simulink model "TwoDOF"  (R2021b)
settings: Solver=VariableStepAuto  StartTime=0.0  StopTime=7  RelTol=1e-3
values from neighbouring files (symbols this model uses):
  Ask = [0 1 0 0 ... (first row only)    [H_inf_ctrl.m]
  Bsk = [0 0 0 0 ... (first row only)    [H_inf_ctrl.m]
  c = 40e3    (= 40000)    [H_inf_ctrl.m]
  c_p = 0.8    [H_inf_ctrl.m]
  c_s = 0.05    [H_inf_ctrl.m]
  c_x = 3300000    [H_inf_ctrl.m]
  c_z = 1000000    [H_inf_ctrl.m]
  Csk = [0 1 0 0 ... (first row only)    [H_inf_ctrl.m]
  Dsk = zeros(2,4)    [H_inf_ctrl.m]
  j = 700e3    (= 700000)    [H_inf_ctrl.m]
  k = 2*300e3    (= 600000)    [H_inf_ctrl.m]
  k_p = 6.32    [H_inf_ctrl.m]
  k_s = 0.0632    [H_inf_ctrl.m]
  L = 6    [H_inf_ctrl.m]
  m = 22000    [H_inf_ctrl.m]
  m_p = 0.16    [H_inf_ctrl.m]
  m_s = 0.16    [H_inf_ctrl.m]
  T = 0.1    [H_inf_ctrl.m]    (also in OneDOF.m = 1.5; PID_Controller.m = 1.5)
  w_n = sqrt(k_p/m_p)    [H_inf_ctrl.m]
undefined symbols (not defined in the file or in its folder): K
settings Model: Creator=thomasperrein  LastModifiedBy=thomasperrein

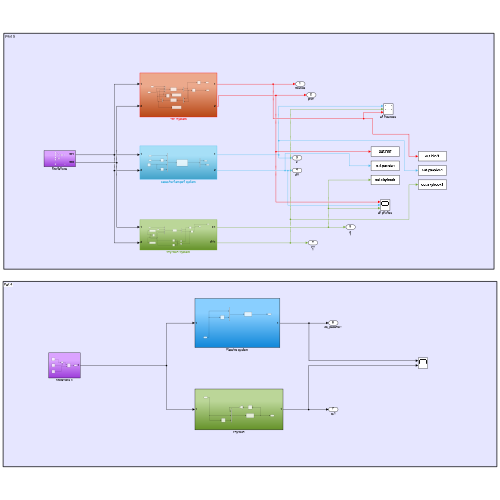
[thumbnail: Simulink's stored preview of the top-level diagram]
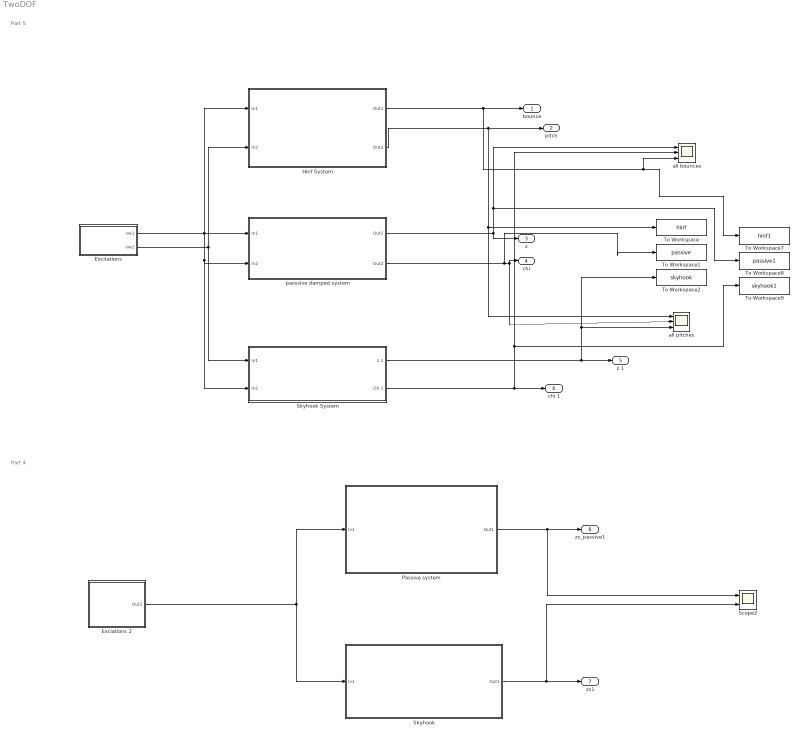
== system TwoDOF ==
  note: Part 4
  note: Part 5
  Exciations 2 : Subsystem
  Excitations : Subsystem
  Hinf System : Subsystem
  Passive system : Subsystem
  Scope2 : Scope  NumInputPorts=2
  Skyhook : Subsystem
  Skyhook System : Subsystem
  To Workspace : ToWorkspace  VariableName=hinf  SaveFormat=Timeseries  SampleTime=-1
  To Workspace1 : ToWorkspace  VariableName=passive  SaveFormat=Timeseries  SampleTime=-1
  To Workspace2 : ToWorkspace  VariableName=skyhook  SaveFormat=Timeseries  SampleTime=-1
  To Workspace7 : ToWorkspace  VariableName=hinf1  SaveFormat=Timeseries  SampleTime=-1
  To Workspace8 : ToWorkspace  VariableName=passive1  SaveFormat=Timeseries  SampleTime=-1
  To Workspace9 : ToWorkspace  VariableName=skyhook1  SaveFormat=Timeseries  SampleTime=-1
  all bounces : Scope  NumInputPorts=3
  all pitches : Scope  NumInputPorts=3
  passsive damped system : Subsystem
  bounce : Outport
  pitch : Outport  Port=2
  "z " : Outport  Port=3  VectorParamsAs1DForOutWhenUnconnected=off
  "chi " : Outport  Port=4  VectorParamsAs1DForOutWhenUnconnected=off
  z 1 : Outport  Port=5  VectorParamsAs1DForOutWhenUnconnected=off
  chi 1 : Outport  Port=6  VectorParamsAs1DForOutWhenUnconnected=off
  zs1 : Outport  Port=7  VectorParamsAs1DForOutWhenUnconnected=off
  zs_passive1 : Outport  Port=8  VectorParamsAs1DForOutWhenUnconnected=off
  wires:
  Skyhook System/1(z 1) -> z 1/1, all pitches/3, To Workspace2/1
  Skyhook System/2(chi 1) -> To Workspace9/1, all bounces/2, chi 1/1
  passsive damped system/2(Out2) -> To Workspace1/1, all pitches/2, "chi "/1
  passsive damped system/1(Out1) -> "z "/1, To Workspace8/1, all bounces/1
  Hinf System/2(Out2) -> all pitches/1, To Workspace/1, pitch/1
  Hinf System/1(Out1) -> bounce/1, To Workspace7/1, all bounces/3
  Excitations/1(sw1) -> Hinf System/1(In1), passsive damped system/1(In1), passsive damped system/2(In2), Skyhook System/2(In2)
  Excitations/2(sw2) -> Hinf System/2(In2), Skyhook System/1(In1)
  Exciations 2/1(Out1) -> Skyhook/1(In1), Passive system/1(In1)
  Passive system/1(Out1) -> zs_passive1/1, Scope2/1
  Skyhook/1(Out1) -> Scope2/2, zs1/1

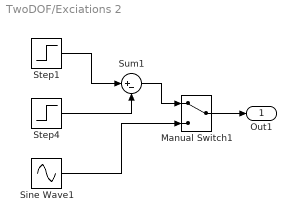
== system TwoDOF/Exciations 2 ==
  Manual Switch1 : ManualSwitch
  Sine Wave1 : Sin  Amplitude=0.05  Frequency=2*pi*w_n  SampleTime=0
  Step1 : Step  Time=0  After=0.05  SampleTime=0
  Step4 : Step  Time=0.1  After=0.05  SampleTime=0
  Sum1 : Sum  Inputs=|+-
  Out1 : Outport
  wires:
  Manual Switch1/1 -> Out1/1
  Step4/1 -> Sum1/2
  Sum1/1 -> Manual Switch1/1
  Sine Wave1/1 -> Manual Switch1/2
  Step1/1 -> Sum1/1

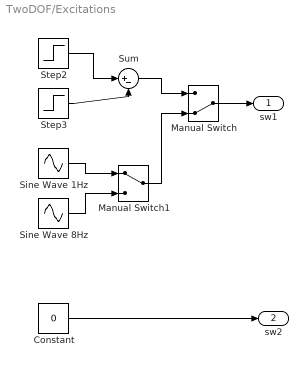
== system TwoDOF/Excitations ==
  Constant : Constant  Value=0
  Manual Switch : ManualSwitch  CurrentSetting=0
  Manual Switch1 : ManualSwitch
  Sine Wave 1Hz : Sin  Amplitude=0.01  Frequency=2*pi*1  SampleTime=0
  Sine Wave 8Hz : Sin  Amplitude=0.01  Frequency=2*pi*8  SampleTime=0
  Step2 : Step  Time=0  After=0.03  SampleTime=0
  Step3 : Step  Time=0.1  After=0.03  SampleTime=0
  Sum : Sum  Inputs=|+-
  sw1 : Outport
  sw2 : Outport  Port=2
  wires:
  Constant/1 -> sw2/1
  Manual Switch/1 -> sw1/1
  Sum/1 -> Manual Switch/1
  Step2/1 -> Sum/1
  Step3/1 -> Sum/2
  Manual Switch1/1 -> Manual Switch/2
  Sine Wave 8Hz/1 -> Manual Switch1/2
  Sine Wave 1Hz/1 -> Manual Switch1/1

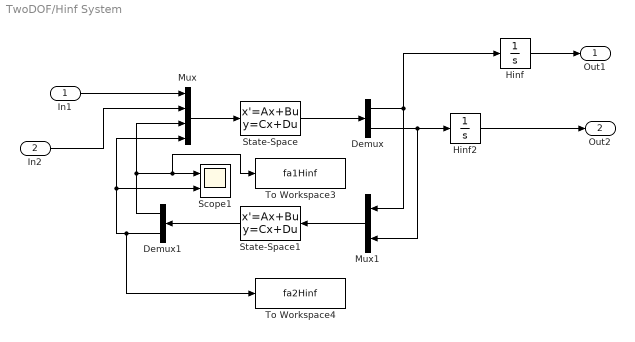
== system TwoDOF/Hinf System ==
  In1 : Inport
  In2 : Inport  Port=2
  Demux : Demux  Outputs=2
  Demux1 : Demux  Outputs=2
  Hinf : Integrator
  Hinf2 : Integrator
  Mux : Mux
  Mux1 : Mux  Inputs=2
  Scope1 : Scope  NumInputPorts=2
  State-Space : StateSpace  A=Ask  B=Bsk  C=Csk  D=Dsk  InitialCondition=0
  State-Space1 : StateSpace  A=K.A  B=K.B  C=K.C  D=K.D  InitialCondition=0
  To Workspace3 : ToWorkspace  VariableName=fa1Hinf  SaveFormat=Timeseries  SampleTime=-1
  To Workspace4 : ToWorkspace  VariableName=fa2Hinf  SaveFormat=Timeseries  SampleTime=-1
  Out1 : Outport
  Out2 : Outport  Port=2
  wires:
  State-Space/1 -> Demux/1
  Hinf/1 -> Out1/1
  Mux1/1 -> State-Space1/1
  State-Space1/1 -> Demux1/1
  Mux/1 -> State-Space/1
  Hinf2/1 -> Out2/1
  In1/1 -> Mux/1
  Demux1/2 -> To Workspace4/1, Mux/4, Scope1/2
  Demux/2 -> Mux1/2, Hinf2/1
  In2/1 -> Mux/2
  Demux1/1 -> Mux/3, To Workspace3/1, Scope1/1
  Demux/1 -> Mux1/1, Hinf/1

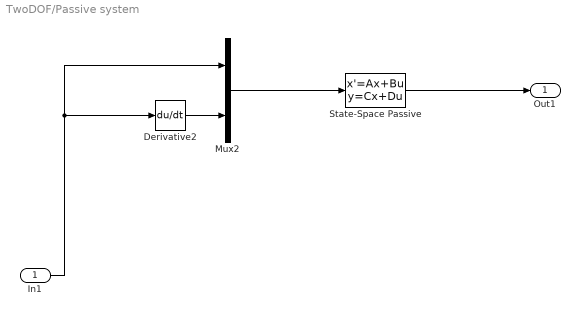
== system TwoDOF/Passive system ==
  In1 : Inport
  Derivative2 : Derivative
  Mux2 : Mux  Inputs=2
  State-Space Passive : StateSpace  A=[0,1,0,0; -k_s/m_s,-c_s/m_s, k_s/m_s,c_s/m_s;0,0,0,1; k_p/m_p,c_s/m_p,-(k_s+k_p)/m_p,-(c_s+c_p)/m_p]  B=[0,0; 0,0; 0,0; k_p/m_p,c_p/m_p]  C=[1,0,0,0]  D=[0,0,]  InitialCondition=[0,0,0,0]
  Out1 : Outport
  wires:
  Derivative2/1 -> Mux2/2
  Mux2/1 -> State-Space Passive/1
  State-Space Passive/1 -> Out1/1
  In1/1 -> Derivative2/1, Mux2/1

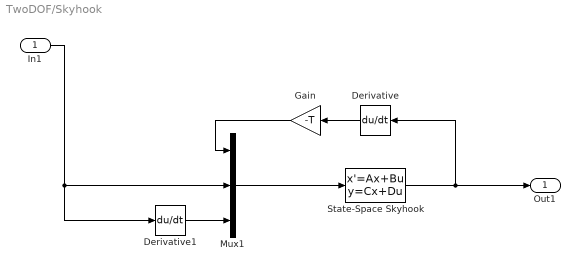
== system TwoDOF/Skyhook ==
  In1 : Inport
  Derivative : Derivative
  Derivative1 : Derivative
  Gain : Gain  Gain=-T
  Mux1 : Mux  Inputs=3
  "State-Space Skyhook " : StateSpace  A=[0,1,0,0; -k_s/m_s,0, k_s/m_s,0;0,0,0,1; k_s/m_p,0,-(k_s+k_p)/m_p,-c_p/m_p]  B=[0,0,0; 1/m_s,0,0; 0,0,0; -1/m_p,k_p/m_p,c_p/m_p]  C=[1,0,0,0]  D=[0,0,0]  InitialCondition=[0,0,0,0]
  Out1 : Outport
  wires:
  Mux1/1 -> "State-Space Skyhook "/1
  Derivative1/1 -> Mux1/3
  Gain/1 -> Mux1/1
  Derivative/1 -> Gain/1
  "State-Space Skyhook "/1 -> Out1/1, Derivative/1
  In1/1 -> Mux1/2, Derivative1/1

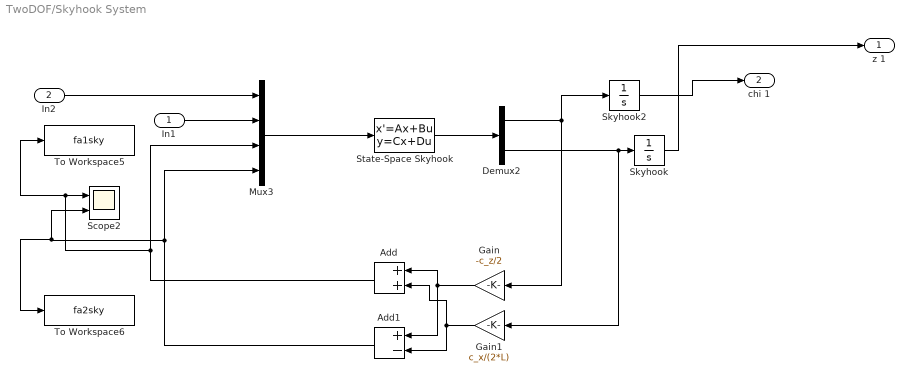
== system TwoDOF/Skyhook System ==
  In1 : Inport
  In2 : Inport  Port=2
  Add : Sum
  Add1 : Sum  Inputs=+-
  Demux2 : Demux  Outputs=2
  Gain : Gain  Gain=-c_z/2
  Gain1 : Gain  Gain=c_x/(2*L)
  Mux3 : Mux
  Scope2 : Scope  NumInputPorts=2
  Skyhook : Integrator
  Skyhook2 : Integrator
  "State-Space Skyhook " : StateSpace  A=[0,1,0,0; 0,0,-2*L*k/m,0; 0,0,0,1; 0,0,-2*k*L^2/j,0]  B=[0,0,0,0; k/m,-k/m,1/m,1/m; 0,0,0,0; k*L/j,-k*L/j,-L/j,L/j]  C=[0,1,0,0; 0,0,0,1]  D=[0,0,0,0; 0,0,0,0]  InitialCondition=[0,0,0,0]
  To Workspace5 : ToWorkspace  VariableName=fa1sky  SaveFormat=Timeseries  SampleTime=-1
  To Workspace6 : ToWorkspace  VariableName=fa2sky  SaveFormat=Timeseries  SampleTime=-1
  z 1 : Outport
  chi 1 : Outport  Port=2
  wires:
  In1/1 -> Mux3/2
  In2/1 -> Mux3/1
  Demux2/1 -> Gain/1, Skyhook2/1
  Demux2/2 -> Gain1/1, Skyhook/1
  Skyhook2/1 -> chi 1/1
  Gain/1 -> Add/1, Add1/1
  Add/1 -> Mux3/3, To Workspace5/1, Scope2/1
  Add1/1 -> Mux3/4, To Workspace6/1, Scope2/2
  Mux3/1 -> "State-Space Skyhook "/1
  Gain1/1 -> Add/2, Add1/2
  Skyhook/1 -> z 1/1
  "State-Space Skyhook "/1 -> Demux2/1

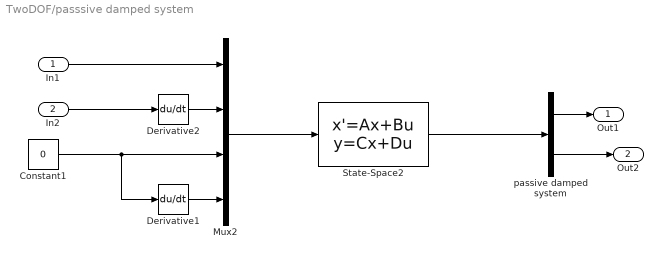
== system TwoDOF/passsive damped system ==
  In1 : Inport
  In2 : Inport  Port=2
  Constant1 : Constant  Value=0
  Derivative1 : Derivative
  Derivative2 : Derivative
  Mux2 : Mux
  State-Space2 : StateSpace  A=[0,1,0,0; 0,0,-2*L*k/m,-2*L*c/m; 0,0,0,1; 0,0,-2*k*L^2/j,-2*c*L^2/j]  B=[0,0,0,0; k/m,c/m,-k/m,-c/m; 0,0,0,0; k*L/j,c*L/j,-k*L/j,-c*L/j]  C=[1,0,0,0; 0,0,1,0]  D=[0,0,0,0; 0,0,0,0]  InitialCondition=[0,0,0,0]
  passive damped system : Demux  Outputs=2
  Out1 : Outport
  Out2 : Outport  Port=2
  wires:
  In2/1 -> Derivative2/1
  passive damped system/2 -> Out2/1
  In1/1 -> Mux2/1
  Derivative1/1 -> Mux2/4
  Mux2/1 -> State-Space2/1
  passive damped system/1 -> Out1/1
  Derivative2/1 -> Mux2/2
  State-Space2/1 -> passive damped system/1
  Constant1/1 -> Derivative1/1, Mux2/3
